simulink model "NonIdealScheme"  (R2021b)
settings: Solver=VariableStepAuto  StartTime=0.0  StopTime=15  RelTol=1e-3
libraries: spsDiodeLib x7, spsMeanLib x6, spsVoltageMeasurementLib x3, spsCurrentMeasurementLib x1, spsDCMachineLib x1, spsDCVoltageSourceLib x1, spsGroundLib x1, spsIGBTLib x1, simulink x1, spsThreePhaseSourceLib x1, spspowerguiLib x1
settings Model: Creator=kkaya674  LastModifiedBy=kkaya674

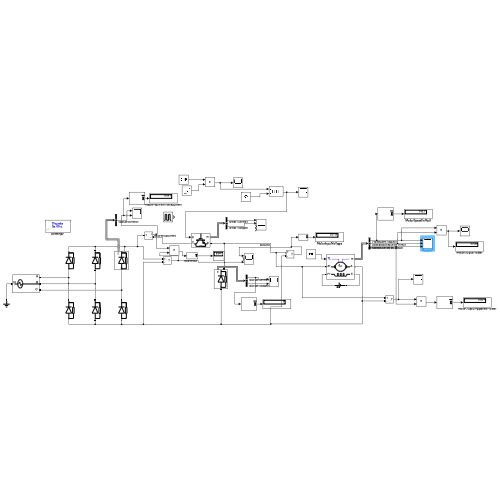
[thumbnail: Simulink's stored preview of the top-level diagram]
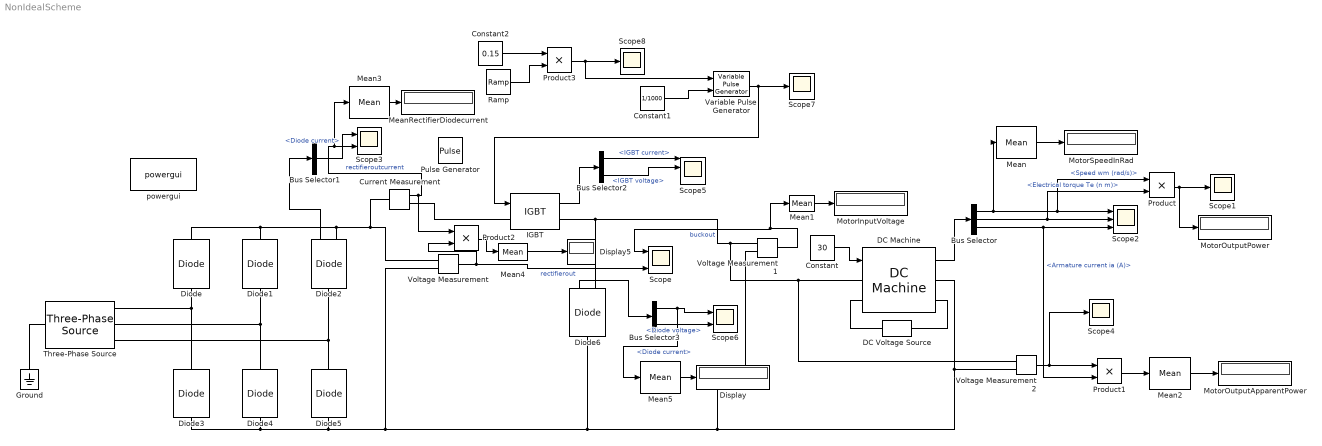
== system NonIdealScheme ==
  Bus Selector : BusSelector  OutputSignals=Speed wm (rad/s),Electrical torque Te (n m),Armature current ia (A)
  Bus Selector1 : BusSelector  OutputSignals=Diode current
  Bus Selector2 : BusSelector  OutputSignals=IGBT current,IGBT voltage
  Bus Selector3 : BusSelector  OutputSignals=Diode current,Diode voltage
  Constant : Constant  Value=30
  Constant1 : Constant  Value=1/1000
  Constant2 : Constant  Value=0.15  VectorParams1D=off
  Current Measurement : spsCurrentMeasurementLib/Current Measurement  PhasorSimulation=off  OutputType=Complex  PSBequivalent=0
  DC Machine : spsDCMachineLib/DC Machine  PresetModel=No  MechanicalLoad=Torque TL  FieldType=Wound  ShowDetailedParameters=on  MeasurementBus=off  RLa=[0.8 12.5e-3]  RLf=[210 23]  Laf=1.8  MachineConstant=Torque constant (N.m/A)  Ke=1.8  Kt=1.8  J=1  Bm=0  Tf=0  w0=0  Ifinit=1.04761904756944  TsPowergui=0  TsBlock=-1
  DC Voltage Source : spsDCVoltageSourceLib/DC Voltage Source  Amplitude=220  Measurements=None
  Diode{,1,3..5} (5 alike) : spsDiodeLib/Diode  Ron=0.001  Lon=0  Vf=0.8  IC=0  UseSnubber=0  Rs=500  Cs=250e-9  Measurements=off
  Diode2 : spsDiodeLib/Diode  Ron=0.001  Lon=0  Vf=0.8  IC=0  UseSnubber=0  Rs=500  Cs=250e-9  Measurements=on
  Diode6 : spsDiodeLib/Diode  Ron=0.001  Lon=0  Vf=0.8  IC=0  UseSnubber=0  Rs=500  Cs=250e-9  Measurements=on
  Display : Display
  Display5 : Display
  Ground : spsGroundLib/Ground  LConnTagsString=a
  IGBT : spsIGBTLib/IGBT  Ron=0.001  Lon=0  Vf=1  Tf=1e-6  Tt=2e-6  IC=0  Rs=1e5  Cs=inf  Measurements=on
  Mean : spsMeanLib/Mean  Freq=60  Vinit=0  Ts=0
  Mean1 : spsMeanLib/Mean  Freq=60  Vinit=0  Ts=0
  Mean2 : spsMeanLib/Mean  Freq=50  Vinit=0  Ts=0
  Mean3 : spsMeanLib/Mean  Freq=50  Vinit=0  Ts=0
  Mean4 : spsMeanLib/Mean  Freq=50  Vinit=0  Ts=0
  Mean5 : spsMeanLib/Mean  Freq=60  Vinit=0  Ts=0
  MeanRectifierDiodecurrent : Display
  MotorInputVoltage : Display
  MotorOutputApparentPower : Display
  MotorOutputPower : Display
  MotorSpeedInRad : Display
  Product{,1..3} (4 alike) : Product
  Pulse Generator : DiscretePulseGenerator  PulseType=Time based  Period=1/1000  PulseWidth=80  VectorParams1D=off
  Ramp : simulink/Sources/Ramp  slope=1  start=0  InitialOutput=0.1
  Scope : Scope  NumInputPorts=3
  Scope{1,4,7..8} (4 alike) : Scope
  Scope2 : Scope  NumInputPorts=3
  Scope3 : Scope  NumInputPorts=2
  Scope5 : Scope  NumInputPorts=4
  Scope6 : Scope  NumInputPorts=2
  Three-Phase Source : spsThreePhaseSourceLib/Three-Phase Source  InternalConnection=Yn  VoltagePhases=off  Voltage=166  PhaseAngle=0  Voltage_phases=[25e3 25e3 25e3]/sqrt(3)  PhaseAngles_phases=[0 -120 +120]  Frequency=50  NonIdealSource=off  SpecifyImpedance=off  Resistance=0.8929  Inductance=16.58e-3  ShortCircuitLevel=100e6  BaseVoltage=25e3  XRratio=7  BusType=swing  Pref=10e3  Qref=0  Prefabc=[10e3, 10e3, 10e3]  Qrefabc=[0, 0, 0]  Qmin=-inf  Qmax=inf
  Variable Pulse Generator : VariablePulseGenerator  AllowZeroPulseWidth=on  SampleTime=0.1
  Voltage Measurement : spsVoltageMeasurementLib/Voltage Measurement  PhasorSimulation=off  OutputType=Complex  PSBequivalent=0
  Voltage Measurement1 : spsVoltageMeasurementLib/Voltage Measurement  PhasorSimulation=off  OutputType=Complex  PSBequivalent=0
  Voltage Measurement2 : spsVoltageMeasurementLib/Voltage Measurement  PhasorSimulation=off  OutputType=Complex  PSBequivalent=0
  powergui : spspowerguiLib/powergui  Priority=1  SimulationMode=Discrete  SampleTime=50e-6  frequency=60  Iterations=50  frequencyindice=0  Pbase=100e6  ErrMax=1e-4  UnitsV=kV  UnitsW=MW  buscounter=0  FunctionMessages=off  echomessages=off  EnableUseOfTLC=off  CurrentSourceSwitches=off  DisableSnubberDevices=off  DisableRonSwitches=off  DisableVfSwitches=off  DisplayEquations=off  AutomaticDiscreteSolvers=off  SolverType=Tustin/Backward Euler (TBE)  Interpol=off  ExternalGateDelay=off  methode=off  Ts=100  x0status=blocks  SPID=on  SwTol=0  HookPort=off  NonlinearTolerance=1e-4  nMaxIteration=100  ContinueOnMaxIteration=off  RestoreLinks=warning  ResistiveCurrentMeasurement=off  Frange=[0:2:500]  Ylog=off  Xlog=on  ShowGrid=off  save=off  variable=ZData  structure=0  ZoomFFT=off  StartTime=0.0  cycles=1  DisplayStyle=1  fundamental=60  FreqAxis=off  MaxFrequency=1000  frequencyindicesteady=1  RmsSteady=1  display=off
  wires:
  Voltage Measurement/1 -> Product2/2, Scope/3  "rectifierout"
  Voltage Measurement1/1 -> Mean1/1, Scope/1  "buckout"
  DC Machine/1 -> Bus Selector/1
  Bus Selector/1 -> Mean/1, Product/1, Scope2/1  "<Speed wm (rad/s)>"
  Mean/1 -> MotorSpeedInRad/1
  Mean1/1 -> MotorInputVoltage/1
  IGBT/1 -> Bus Selector2/1
  Bus Selector2/1 -> Scope5/1  "<IGBT current>"
  Bus Selector2/2 -> Scope5/2  "<IGBT voltage>"
  Diode6/1 -> Bus Selector3/1
  Bus Selector3/1 -> Mean5/1, Scope6/1  "<Diode current>"
  Bus Selector3/2 -> Scope6/2  "<Diode voltage>"
  Constant/1 -> DC Machine/1
  Product/1 -> MotorOutputPower/1, Scope1/1
  Voltage Measurement2/1 -> Product1/1, Scope4/1
  Bus Selector/3 -> Product1/2, Scope2/3  "<Armature current ia (A)>"
  Bus Selector/2 -> Product/2, Scope2/2  "<Electrical torque Te (n m)>"
  Product1/1 -> Mean2/1
  Mean2/1 -> MotorOutputApparentPower/1
  Diode2/1 -> Bus Selector1/1
  Bus Selector1/1 -> Scope3/1  "<Diode current>"
  Current Measurement/1 -> Product2/1, Mean3/1, Scope3/2  "rectifieroutcurrent"
  Mean3/1 -> MeanRectifierDiodecurrent/1
  Product2/1 -> Mean4/1
  Mean4/1 -> Display5/1
  Mean5/1 -> Display/1
  Constant2/1 -> Product3/1
  Ramp/1 -> Product3/2
  Product3/1 -> Variable Pulse Generator/1, Scope8/1
  Constant1/1 -> Variable Pulse Generator/2
  Variable Pulse Generator/1 -> IGBT/1, Scope7/1
  connections:
  Three-Phase Source/RConn1 -- Diode/LConn1 -- Diode3/RConn1
  Three-Phase Source/RConn2 -- Diode1/LConn1 -- Diode4/RConn1
  Three-Phase Source/RConn3 -- Diode5/RConn1 -- Diode2/LConn1
  Diode4/LConn1 -- Diode3/LConn1 -- Voltage Measurement/LConn2 -- Voltage Measurement2/LConn2 -- DC Machine/RConn1 -- Voltage Measurement1/LConn2 -- Diode6/LConn1 -- Diode5/LConn1
  Diode/RConn1 -- Voltage Measurement/LConn1 -- Current Measurement/LConn1 -- Diode2/RConn1 -- Diode1/RConn1
  Three-Phase Source/LConn1 -- Ground/LConn1
  DC Voltage Source/RConn1 -- DC Machine/LConn2
  DC Voltage Source/LConn1 -- DC Machine/RConn2
  Voltage Measurement1/LConn1 -- Voltage Measurement2/LConn1 -- DC Machine/LConn1 -- IGBT/RConn1 -- Diode6/RConn1
  IGBT/LConn1 -- Current Measurement/RConn1
